simulink model "gm_test_prediction_without_delays"  (R2022a)
settings: Solver=FixedStepDiscrete  StartTime=0.0  StopTime=10.0  RelTol=1e-3
undefined symbols (not defined in the file or in its folder): f_c, L_d, L_q, L_x, L_y, p, psi_pm, R_ph
libraries: hdlmdlgenlib x2
(part 7 of 9)

== system gm_test_prediction_without_delays/Prediction_and_cost_function1/Subsystem/Subsystem12/Add2 ==
  In1 : Inport
  In2 : Inport  Port=2
  Add2 : Sum  OutDataTypeStr=single  SampleTime=1e-08
  Add2_pd1 : Delay  DelayLength=6
  Out1 : Outport
  wires:
  In1/1 -> Add2/1
  In2/1 -> Add2/2
  Add2/1 -> Add2_pd1/1
  Add2_pd1/1 -> Out1/1

== system gm_test_prediction_without_delays/Prediction_and_cost_function1/Subsystem/Subsystem12/Add3 ==
  In1 : Inport
  In2 : Inport  Port=2
  Add3 : Sum  OutDataTypeStr=single  SampleTime=1e-08
  Add3_pd1 : Delay  DelayLength=6
  Out1 : Outport
  wires:
  In1/1 -> Add3/1
  In2/1 -> Add3/2
  Add3/1 -> Add3_pd1/1
  Add3_pd1/1 -> Out1/1

== system gm_test_prediction_without_delays/Prediction_and_cost_function1/Subsystem/Subsystem12/Add4 ==
  In1 : Inport
  In2 : Inport  Port=2
  Add4 : Sum  OutDataTypeStr=single  SampleTime=1e-08
  Add4_pd1 : Delay  DelayLength=6
  Out1 : Outport
  wires:
  In1/1 -> Add4/1
  In2/1 -> Add4/2
  Add4/1 -> Add4_pd1/1
  Add4_pd1/1 -> Out1/1

== system gm_test_prediction_without_delays/Prediction_and_cost_function1/Subsystem/Subsystem12/Product1 ==
  In1 : Inport
  In2 : Inport  Port=2
  Product1 : Product  Inputs=**  OutDataTypeStr=single  SampleTime=1e-08
  Product1_pd1 : Delay  DelayLength=6
  Out1 : Outport
  wires:
  In1/1 -> Product1/1
  In2/1 -> Product1/2
  Product1/1 -> Product1_pd1/1
  Product1_pd1/1 -> Out1/1

== system gm_test_prediction_without_delays/Prediction_and_cost_function1/Subsystem/Subsystem12/Product10 ==
  In1 : Inport
  In2 : Inport  Port=2
  Product10 : Product  Inputs=**  OutDataTypeStr=single  SampleTime=1e-08
  Product10_pd1 : Delay  DelayLength=6
  Out1 : Outport
  wires:
  In1/1 -> Product10/1
  In2/1 -> Product10/2
  Product10/1 -> Product10_pd1/1
  Product10_pd1/1 -> Out1/1

== system gm_test_prediction_without_delays/Prediction_and_cost_function1/Subsystem/Subsystem12/Product11 ==
  In1 : Inport
  In2 : Inport  Port=2
  Product11 : Product  Inputs=**  OutDataTypeStr=single  SampleTime=1e-08
  Product11_pd1 : Delay  DelayLength=6
  Out1 : Outport
  wires:
  In1/1 -> Product11/1
  In2/1 -> Product11/2
  Product11/1 -> Product11_pd1/1
  Product11_pd1/1 -> Out1/1

== system gm_test_prediction_without_delays/Prediction_and_cost_function1/Subsystem/Subsystem12/Product2 ==
  In1 : Inport
  In2 : Inport  Port=2
  Product2 : Product  Inputs=**  OutDataTypeStr=single  SampleTime=1e-08
  Product2_pd1 : Delay  DelayLength=6
  Out1 : Outport
  wires:
  In1/1 -> Product2/1
  In2/1 -> Product2/2
  Product2/1 -> Product2_pd1/1
  Product2_pd1/1 -> Out1/1

== system gm_test_prediction_without_delays/Prediction_and_cost_function1/Subsystem/Subsystem12/Product3 ==
  In1 : Inport
  In2 : Inport  Port=2
  Product3 : Product  Inputs=**  OutDataTypeStr=single  SampleTime=1e-08
  Product3_pd1 : Delay  DelayLength=6
  Out1 : Outport
  wires:
  In1/1 -> Product3/1
  In2/1 -> Product3/2
  Product3/1 -> Product3_pd1/1
  Product3_pd1/1 -> Out1/1

== system gm_test_prediction_without_delays/Prediction_and_cost_function1/Subsystem/Subsystem12/Product31 ==
  In1 : Inport
  In2 : Inport  Port=2
  Product31 : Product  Inputs=**  OutDataTypeStr=single  SampleTime=1e-08
  Product31_pd1 : Delay  DelayLength=6
  Out1 : Outport
  wires:
  In1/1 -> Product31/1
  In2/1 -> Product31/2
  Product31/1 -> Product31_pd1/1
  Product31_pd1/1 -> Out1/1

== system gm_test_prediction_without_delays/Prediction_and_cost_function1/Subsystem/Subsystem12/Product4 ==
  In1 : Inport
  In2 : Inport  Port=2
  Product4 : Product  Inputs=**  OutDataTypeStr=single  SampleTime=1e-08
  Product4_pd1 : Delay  DelayLength=6
  Out1 : Outport
  wires:
  In1/1 -> Product4/1
  In2/1 -> Product4/2
  Product4/1 -> Product4_pd1/1
  Product4_pd1/1 -> Out1/1

== system gm_test_prediction_without_delays/Prediction_and_cost_function1/Subsystem/Subsystem12/Product5 ==
  In1 : Inport
  In2 : Inport  Port=2
  Product5 : Product  Inputs=**  OutDataTypeStr=single  SampleTime=1e-08
  Product5_pd1 : Delay  DelayLength=6
  Out1 : Outport
  wires:
  In1/1 -> Product5/1
  In2/1 -> Product5/2
  Product5/1 -> Product5_pd1/1
  Product5_pd1/1 -> Out1/1

== system gm_test_prediction_without_delays/Prediction_and_cost_function1/Subsystem/Subsystem12/Product6 ==
  In1 : Inport
  In2 : Inport  Port=2
  Product6 : Product  Inputs=**  OutDataTypeStr=single  SampleTime=1e-08
  Product6_pd1 : Delay  DelayLength=6
  Out1 : Outport
  wires:
  In1/1 -> Product6/1
  In2/1 -> Product6/2
  Product6/1 -> Product6_pd1/1
  Product6_pd1/1 -> Out1/1

== system gm_test_prediction_without_delays/Prediction_and_cost_function1/Subsystem/Subsystem12/Product7 ==
  In1 : Inport
  In2 : Inport  Port=2
  Product7 : Product  Inputs=**  OutDataTypeStr=single  SampleTime=1e-08
  Product7_pd1 : Delay  DelayLength=6
  Out1 : Outport
  wires:
  In1/1 -> Product7/1
  In2/1 -> Product7/2
  Product7/1 -> Product7_pd1/1
  Product7_pd1/1 -> Out1/1

== system gm_test_prediction_without_delays/Prediction_and_cost_function1/Subsystem/Subsystem12/Product8 ==
  In1 : Inport
  In2 : Inport  Port=2
  Product8 : Product  Inputs=**  OutDataTypeStr=single  SampleTime=1e-08
  Product8_pd1 : Delay  DelayLength=6
  Out1 : Outport
  wires:
  In1/1 -> Product8/1
  In2/1 -> Product8/2
  Product8/1 -> Product8_pd1/1
  Product8_pd1/1 -> Out1/1

== system gm_test_prediction_without_delays/Prediction_and_cost_function1/Subsystem/Subsystem12/Product9 ==
  In1 : Inport
  In2 : Inport  Port=2
  Product9 : Product  Inputs=**  OutDataTypeStr=single  SampleTime=1e-08
  Product9_pd1 : Delay  DelayLength=6
  Out1 : Outport
  wires:
  In1/1 -> Product9/1
  In2/1 -> Product9/2
  Product9/1 -> Product9_pd1/1
  Product9_pd1/1 -> Out1/1

== system gm_test_prediction_without_delays/Prediction_and_cost_function1/Subsystem/Subsystem12/Subtract1_stage2 ==
  In1 : Inport
  In2 : Inport  Port=2
  Subtract1_stage2 : Sum  Inputs=+-  OutDataTypeStr=single  SampleTime=1e-08
  Subtract1_stage2_pd1 : Delay  DelayLength=6
  Out1 : Outport
  wires:
  In1/1 -> Subtract1_stage2/1
  In2/1 -> Subtract1_stage2/2
  Subtract1_stage2/1 -> Subtract1_stage2_pd1/1
  Subtract1_stage2_pd1/1 -> Out1/1

== system gm_test_prediction_without_delays/Prediction_and_cost_function1/Subsystem/Subsystem12/Subtract1_stage3 ==
  In1 : Inport
  In2 : Inport  Port=2
  Subtract1_stage3 : Sum  Inputs=+-  OutDataTypeStr=single  SampleTime=1e-08
  Subtract1_stage3_pd1 : Delay  DelayLength=6
  Out1 : Outport
  wires:
  In1/1 -> Subtract1_stage3/1
  In2/1 -> Subtract1_stage3/2
  Subtract1_stage3/1 -> Subtract1_stage3_pd1/1
  Subtract1_stage3_pd1/1 -> Out1/1

== system gm_test_prediction_without_delays/Prediction_and_cost_function1/Subsystem/Subsystem12/Subtract2 ==
  In1 : Inport
  In2 : Inport  Port=2
  Subtract2 : Sum  Inputs=+-  OutDataTypeStr=single  SampleTime=1e-08
  Subtract2_pd1 : Delay  DelayLength=6
  Out1 : Outport
  wires:
  In1/1 -> Subtract2/1
  In2/1 -> Subtract2/2
  Subtract2/1 -> Subtract2_pd1/1
  Subtract2_pd1/1 -> Out1/1

== system gm_test_prediction_without_delays/Prediction_and_cost_function1/Subsystem/Subsystem12/Subtract3 ==
  In1 : Inport
  In2 : Inport  Port=2
  Subtract3 : Sum  Inputs=+-  OutDataTypeStr=single  SampleTime=1e-08
  Subtract3_pd1 : Delay  DelayLength=6
  Out1 : Outport
  wires:
  In1/1 -> Subtract3/1
  In2/1 -> Subtract3/2
  Subtract3/1 -> Subtract3_pd1/1
  Subtract3_pd1/1 -> Out1/1

== system gm_test_prediction_without_delays/Prediction_and_cost_function1/Subsystem/Subsystem12/Subtract_stage2 ==
  In1 : Inport
  In2 : Inport  Port=2
  Subtract_stage2 : Sum  Inputs=+-  OutDataTypeStr=single  SampleTime=1e-08
  Subtract_stage2_pd1 : Delay  DelayLength=6
  Out1 : Outport
  wires:
  In1/1 -> Subtract_stage2/1
  In2/1 -> Subtract_stage2/2
  Subtract_stage2/1 -> Subtract_stage2_pd1/1
  Subtract_stage2_pd1/1 -> Out1/1

== system gm_test_prediction_without_delays/Prediction_and_cost_function1/Subsystem/Subsystem12/Subtract_stage3 ==
  In1 : Inport
  In2 : Inport  Port=2
  Subtract_stage3 : Sum  OutDataTypeStr=single  SampleTime=1e-08
  Subtract_stage3_pd1 : Delay  DelayLength=6
  Out1 : Outport
  wires:
  In1/1 -> Subtract_stage3/1
  In2/1 -> Subtract_stage3/2
  Subtract_stage3/1 -> Subtract_stage3_pd1/1
  Subtract_stage3_pd1/1 -> Out1/1

== system gm_test_prediction_without_delays/Prediction_and_cost_function1/Subsystem/Subsystem13/Add ==
  In1 : Inport
  In2 : Inport  Port=2
  Add : Sum  OutDataTypeStr=single  SampleTime=1e-08
  Add_pd1 : Delay  DelayLength=6
  Out1 : Outport
  wires:
  In1/1 -> Add/1
  In2/1 -> Add/2
  Add/1 -> Add_pd1/1
  Add_pd1/1 -> Out1/1

== system gm_test_prediction_without_delays/Prediction_and_cost_function1/Subsystem/Subsystem13/Add1 ==
  In1 : Inport
  In2 : Inport  Port=2
  Add1 : Sum  OutDataTypeStr=single  SampleTime=1e-08
  Add1_pd1 : Delay  DelayLength=6
  Out1 : Outport
  wires:
  In1/1 -> Add1/1
  In2/1 -> Add1/2
  Add1/1 -> Add1_pd1/1
  Add1_pd1/1 -> Out1/1

== system gm_test_prediction_without_delays/Prediction_and_cost_function1/Subsystem/Subsystem13/Add2 ==
  In1 : Inport
  In2 : Inport  Port=2
  Add2 : Sum  OutDataTypeStr=single  SampleTime=1e-08
  Add2_pd1 : Delay  DelayLength=6
  Out1 : Outport
  wires:
  In1/1 -> Add2/1
  In2/1 -> Add2/2
  Add2/1 -> Add2_pd1/1
  Add2_pd1/1 -> Out1/1

== system gm_test_prediction_without_delays/Prediction_and_cost_function1/Subsystem/Subsystem13/Add3 ==
  In1 : Inport
  In2 : Inport  Port=2
  Add3 : Sum  OutDataTypeStr=single  SampleTime=1e-08
  Add3_pd1 : Delay  DelayLength=6
  Out1 : Outport
  wires:
  In1/1 -> Add3/1
  In2/1 -> Add3/2
  Add3/1 -> Add3_pd1/1
  Add3_pd1/1 -> Out1/1

== system gm_test_prediction_without_delays/Prediction_and_cost_function1/Subsystem/Subsystem13/Add4 ==
  In1 : Inport
  In2 : Inport  Port=2
  Add4 : Sum  OutDataTypeStr=single  SampleTime=1e-08
  Add4_pd1 : Delay  DelayLength=6
  Out1 : Outport
  wires:
  In1/1 -> Add4/1
  In2/1 -> Add4/2
  Add4/1 -> Add4_pd1/1
  Add4_pd1/1 -> Out1/1

== system gm_test_prediction_without_delays/Prediction_and_cost_function1/Subsystem/Subsystem13/Product1 ==
  In1 : Inport
  In2 : Inport  Port=2
  Product1 : Product  Inputs=**  OutDataTypeStr=single  SampleTime=1e-08
  Product1_pd1 : Delay  DelayLength=6
  Out1 : Outport
  wires:
  In1/1 -> Product1/1
  In2/1 -> Product1/2
  Product1/1 -> Product1_pd1/1
  Product1_pd1/1 -> Out1/1

== system gm_test_prediction_without_delays/Prediction_and_cost_function1/Subsystem/Subsystem13/Product10 ==
  In1 : Inport
  In2 : Inport  Port=2
  Product10 : Product  Inputs=**  OutDataTypeStr=single  SampleTime=1e-08
  Product10_pd1 : Delay  DelayLength=6
  Out1 : Outport
  wires:
  In1/1 -> Product10/1
  In2/1 -> Product10/2
  Product10/1 -> Product10_pd1/1
  Product10_pd1/1 -> Out1/1

== system gm_test_prediction_without_delays/Prediction_and_cost_function1/Subsystem/Subsystem13/Product11 ==
  In1 : Inport
  In2 : Inport  Port=2
  Product11 : Product  Inputs=**  OutDataTypeStr=single  SampleTime=1e-08
  Product11_pd1 : Delay  DelayLength=6
  Out1 : Outport
  wires:
  In1/1 -> Product11/1
  In2/1 -> Product11/2
  Product11/1 -> Product11_pd1/1
  Product11_pd1/1 -> Out1/1

== system gm_test_prediction_without_delays/Prediction_and_cost_function1/Subsystem/Subsystem13/Product2 ==
  In1 : Inport
  In2 : Inport  Port=2
  Product2 : Product  Inputs=**  OutDataTypeStr=single  SampleTime=1e-08
  Product2_pd1 : Delay  DelayLength=6
  Out1 : Outport
  wires:
  In1/1 -> Product2/1
  In2/1 -> Product2/2
  Product2/1 -> Product2_pd1/1
  Product2_pd1/1 -> Out1/1

== system gm_test_prediction_without_delays/Prediction_and_cost_function1/Subsystem/Subsystem13/Product3 ==
  In1 : Inport
  In2 : Inport  Port=2
  Product3 : Product  Inputs=**  OutDataTypeStr=single  SampleTime=1e-08
  Product3_pd1 : Delay  DelayLength=6
  Out1 : Outport
  wires:
  In1/1 -> Product3/1
  In2/1 -> Product3/2
  Product3/1 -> Product3_pd1/1
  Product3_pd1/1 -> Out1/1

== system gm_test_prediction_without_delays/Prediction_and_cost_function1/Subsystem/Subsystem13/Product31 ==
  In1 : Inport
  In2 : Inport  Port=2
  Product31 : Product  Inputs=**  OutDataTypeStr=single  SampleTime=1e-08
  Product31_pd1 : Delay  DelayLength=6
  Out1 : Outport
  wires:
  In1/1 -> Product31/1
  In2/1 -> Product31/2
  Product31/1 -> Product31_pd1/1
  Product31_pd1/1 -> Out1/1

== system gm_test_prediction_without_delays/Prediction_and_cost_function1/Subsystem/Subsystem13/Product4 ==
  In1 : Inport
  In2 : Inport  Port=2
  Product4 : Product  Inputs=**  OutDataTypeStr=single  SampleTime=1e-08
  Product4_pd1 : Delay  DelayLength=6
  Out1 : Outport
  wires:
  In1/1 -> Product4/1
  In2/1 -> Product4/2
  Product4/1 -> Product4_pd1/1
  Product4_pd1/1 -> Out1/1

== system gm_test_prediction_without_delays/Prediction_and_cost_function1/Subsystem/Subsystem13/Product5 ==
  In1 : Inport
  In2 : Inport  Port=2
  Product5 : Product  Inputs=**  OutDataTypeStr=single  SampleTime=1e-08
  Product5_pd1 : Delay  DelayLength=6
  Out1 : Outport
  wires:
  In1/1 -> Product5/1
  In2/1 -> Product5/2
  Product5/1 -> Product5_pd1/1
  Product5_pd1/1 -> Out1/1

== system gm_test_prediction_without_delays/Prediction_and_cost_function1/Subsystem/Subsystem13/Product6 ==
  In1 : Inport
  In2 : Inport  Port=2
  Product6 : Product  Inputs=**  OutDataTypeStr=single  SampleTime=1e-08
  Product6_pd1 : Delay  DelayLength=6
  Out1 : Outport
  wires:
  In1/1 -> Product6/1
  In2/1 -> Product6/2
  Product6/1 -> Product6_pd1/1
  Product6_pd1/1 -> Out1/1

== system gm_test_prediction_without_delays/Prediction_and_cost_function1/Subsystem/Subsystem13/Product7 ==
  In1 : Inport
  In2 : Inport  Port=2
  Product7 : Product  Inputs=**  OutDataTypeStr=single  SampleTime=1e-08
  Product7_pd1 : Delay  DelayLength=6
  Out1 : Outport
  wires:
  In1/1 -> Product7/1
  In2/1 -> Product7/2
  Product7/1 -> Product7_pd1/1
  Product7_pd1/1 -> Out1/1

== system gm_test_prediction_without_delays/Prediction_and_cost_function1/Subsystem/Subsystem13/Product8 ==
  In1 : Inport
  In2 : Inport  Port=2
  Product8 : Product  Inputs=**  OutDataTypeStr=single  SampleTime=1e-08
  Product8_pd1 : Delay  DelayLength=6
  Out1 : Outport
  wires:
  In1/1 -> Product8/1
  In2/1 -> Product8/2
  Product8/1 -> Product8_pd1/1
  Product8_pd1/1 -> Out1/1

== system gm_test_prediction_without_delays/Prediction_and_cost_function1/Subsystem/Subsystem13/Product9 ==
  In1 : Inport
  In2 : Inport  Port=2
  Product9 : Product  Inputs=**  OutDataTypeStr=single  SampleTime=1e-08
  Product9_pd1 : Delay  DelayLength=6
  Out1 : Outport
  wires:
  In1/1 -> Product9/1
  In2/1 -> Product9/2
  Product9/1 -> Product9_pd1/1
  Product9_pd1/1 -> Out1/1

== system gm_test_prediction_without_delays/Prediction_and_cost_function1/Subsystem/Subsystem13/Subtract1_stage2 ==
  In1 : Inport
  In2 : Inport  Port=2
  Subtract1_stage2 : Sum  Inputs=+-  OutDataTypeStr=single  SampleTime=1e-08
  Subtract1_stage2_pd1 : Delay  DelayLength=6
  Out1 : Outport
  wires:
  In1/1 -> Subtract1_stage2/1
  In2/1 -> Subtract1_stage2/2
  Subtract1_stage2/1 -> Subtract1_stage2_pd1/1
  Subtract1_stage2_pd1/1 -> Out1/1

== system gm_test_prediction_without_delays/Prediction_and_cost_function1/Subsystem/Subsystem13/Subtract1_stage3 ==
  In1 : Inport
  In2 : Inport  Port=2
  Subtract1_stage3 : Sum  Inputs=+-  OutDataTypeStr=single  SampleTime=1e-08
  Subtract1_stage3_pd1 : Delay  DelayLength=6
  Out1 : Outport
  wires:
  In1/1 -> Subtract1_stage3/1
  In2/1 -> Subtract1_stage3/2
  Subtract1_stage3/1 -> Subtract1_stage3_pd1/1
  Subtract1_stage3_pd1/1 -> Out1/1

== system gm_test_prediction_without_delays/Prediction_and_cost_function1/Subsystem/Subsystem13/Subtract2 ==
  In1 : Inport
  In2 : Inport  Port=2
  Subtract2 : Sum  Inputs=+-  OutDataTypeStr=single  SampleTime=1e-08
  Subtract2_pd1 : Delay  DelayLength=6
  Out1 : Outport
  wires:
  In1/1 -> Subtract2/1
  In2/1 -> Subtract2/2
  Subtract2/1 -> Subtract2_pd1/1
  Subtract2_pd1/1 -> Out1/1

== system gm_test_prediction_without_delays/Prediction_and_cost_function1/Subsystem/Subsystem13/Subtract3 ==
  In1 : Inport
  In2 : Inport  Port=2
  Subtract3 : Sum  Inputs=+-  OutDataTypeStr=single  SampleTime=1e-08
  Subtract3_pd1 : Delay  DelayLength=6
  Out1 : Outport
  wires:
  In1/1 -> Subtract3/1
  In2/1 -> Subtract3/2
  Subtract3/1 -> Subtract3_pd1/1
  Subtract3_pd1/1 -> Out1/1

== system gm_test_prediction_without_delays/Prediction_and_cost_function1/Subsystem/Subsystem13/Subtract_stage2 ==
  In1 : Inport
  In2 : Inport  Port=2
  Subtract_stage2 : Sum  Inputs=+-  OutDataTypeStr=single  SampleTime=1e-08
  Subtract_stage2_pd1 : Delay  DelayLength=6
  Out1 : Outport
  wires:
  In1/1 -> Subtract_stage2/1
  In2/1 -> Subtract_stage2/2
  Subtract_stage2/1 -> Subtract_stage2_pd1/1
  Subtract_stage2_pd1/1 -> Out1/1

== system gm_test_prediction_without_delays/Prediction_and_cost_function1/Subsystem/Subsystem13/Subtract_stage3 ==
  In1 : Inport
  In2 : Inport  Port=2
  Subtract_stage3 : Sum  OutDataTypeStr=single  SampleTime=1e-08
  Subtract_stage3_pd1 : Delay  DelayLength=6
  Out1 : Outport
  wires:
  In1/1 -> Subtract_stage3/1
  In2/1 -> Subtract_stage3/2
  Subtract_stage3/1 -> Subtract_stage3_pd1/1
  Subtract_stage3_pd1/1 -> Out1/1

== system gm_test_prediction_without_delays/Prediction_and_cost_function1/Subsystem/Subsystem14/Add ==
  In1 : Inport
  In2 : Inport  Port=2
  Add : Sum  OutDataTypeStr=single  SampleTime=1e-08
  Add_pd1 : Delay  DelayLength=6
  Out1 : Outport
  wires:
  In1/1 -> Add/1
  In2/1 -> Add/2
  Add/1 -> Add_pd1/1
  Add_pd1/1 -> Out1/1

== system gm_test_prediction_without_delays/Prediction_and_cost_function1/Subsystem/Subsystem14/Add1 ==
  In1 : Inport
  In2 : Inport  Port=2
  Add1 : Sum  OutDataTypeStr=single  SampleTime=1e-08
  Add1_pd1 : Delay  DelayLength=6
  Out1 : Outport
  wires:
  In1/1 -> Add1/1
  In2/1 -> Add1/2
  Add1/1 -> Add1_pd1/1
  Add1_pd1/1 -> Out1/1

== system gm_test_prediction_without_delays/Prediction_and_cost_function1/Subsystem/Subsystem14/Add2 ==
  In1 : Inport
  In2 : Inport  Port=2
  Add2 : Sum  OutDataTypeStr=single  SampleTime=1e-08
  Add2_pd1 : Delay  DelayLength=6
  Out1 : Outport
  wires:
  In1/1 -> Add2/1
  In2/1 -> Add2/2
  Add2/1 -> Add2_pd1/1
  Add2_pd1/1 -> Out1/1

== system gm_test_prediction_without_delays/Prediction_and_cost_function1/Subsystem/Subsystem14/Add3 ==
  In1 : Inport
  In2 : Inport  Port=2
  Add3 : Sum  OutDataTypeStr=single  SampleTime=1e-08
  Add3_pd1 : Delay  DelayLength=6
  Out1 : Outport
  wires:
  In1/1 -> Add3/1
  In2/1 -> Add3/2
  Add3/1 -> Add3_pd1/1
  Add3_pd1/1 -> Out1/1

== system gm_test_prediction_without_delays/Prediction_and_cost_function1/Subsystem/Subsystem14/Add4 ==
  In1 : Inport
  In2 : Inport  Port=2
  Add4 : Sum  OutDataTypeStr=single  SampleTime=1e-08
  Add4_pd1 : Delay  DelayLength=6
  Out1 : Outport
  wires:
  In1/1 -> Add4/1
  In2/1 -> Add4/2
  Add4/1 -> Add4_pd1/1
  Add4_pd1/1 -> Out1/1

== system gm_test_prediction_without_delays/Prediction_and_cost_function1/Subsystem/Subsystem14/Product1 ==
  In1 : Inport
  In2 : Inport  Port=2
  Product1 : Product  Inputs=**  OutDataTypeStr=single  SampleTime=1e-08
  Product1_pd1 : Delay  DelayLength=6
  Out1 : Outport
  wires:
  In1/1 -> Product1/1
  In2/1 -> Product1/2
  Product1/1 -> Product1_pd1/1
  Product1_pd1/1 -> Out1/1

== system gm_test_prediction_without_delays/Prediction_and_cost_function1/Subsystem/Subsystem14/Product10 ==
  In1 : Inport
  In2 : Inport  Port=2
  Product10 : Product  Inputs=**  OutDataTypeStr=single  SampleTime=1e-08
  Product10_pd1 : Delay  DelayLength=6
  Out1 : Outport
  wires:
  In1/1 -> Product10/1
  In2/1 -> Product10/2
  Product10/1 -> Product10_pd1/1
  Product10_pd1/1 -> Out1/1

== system gm_test_prediction_without_delays/Prediction_and_cost_function1/Subsystem/Subsystem14/Product11 ==
  In1 : Inport
  In2 : Inport  Port=2
  Product11 : Product  Inputs=**  OutDataTypeStr=single  SampleTime=1e-08
  Product11_pd1 : Delay  DelayLength=6
  Out1 : Outport
  wires:
  In1/1 -> Product11/1
  In2/1 -> Product11/2
  Product11/1 -> Product11_pd1/1
  Product11_pd1/1 -> Out1/1

== system gm_test_prediction_without_delays/Prediction_and_cost_function1/Subsystem/Subsystem14/Product2 ==
  In1 : Inport
  In2 : Inport  Port=2
  Product2 : Product  Inputs=**  OutDataTypeStr=single  SampleTime=1e-08
  Product2_pd1 : Delay  DelayLength=6
  Out1 : Outport
  wires:
  In1/1 -> Product2/1
  In2/1 -> Product2/2
  Product2/1 -> Product2_pd1/1
  Product2_pd1/1 -> Out1/1

== system gm_test_prediction_without_delays/Prediction_and_cost_function1/Subsystem/Subsystem14/Product3 ==
  In1 : Inport
  In2 : Inport  Port=2
  Product3 : Product  Inputs=**  OutDataTypeStr=single  SampleTime=1e-08
  Product3_pd1 : Delay  DelayLength=6
  Out1 : Outport
  wires:
  In1/1 -> Product3/1
  In2/1 -> Product3/2
  Product3/1 -> Product3_pd1/1
  Product3_pd1/1 -> Out1/1

== system gm_test_prediction_without_delays/Prediction_and_cost_function1/Subsystem/Subsystem14/Product31 ==
  In1 : Inport
  In2 : Inport  Port=2
  Product31 : Product  Inputs=**  OutDataTypeStr=single  SampleTime=1e-08
  Product31_pd1 : Delay  DelayLength=6
  Out1 : Outport
  wires:
  In1/1 -> Product31/1
  In2/1 -> Product31/2
  Product31/1 -> Product31_pd1/1
  Product31_pd1/1 -> Out1/1

== system gm_test_prediction_without_delays/Prediction_and_cost_function1/Subsystem/Subsystem14/Product4 ==
  In1 : Inport
  In2 : Inport  Port=2
  Product4 : Product  Inputs=**  OutDataTypeStr=single  SampleTime=1e-08
  Product4_pd1 : Delay  DelayLength=6
  Out1 : Outport
  wires:
  In1/1 -> Product4/1
  In2/1 -> Product4/2
  Product4/1 -> Product4_pd1/1
  Product4_pd1/1 -> Out1/1

== system gm_test_prediction_without_delays/Prediction_and_cost_function1/Subsystem/Subsystem14/Product5 ==
  In1 : Inport
  In2 : Inport  Port=2
  Product5 : Product  Inputs=**  OutDataTypeStr=single  SampleTime=1e-08
  Product5_pd1 : Delay  DelayLength=6
  Out1 : Outport
  wires:
  In1/1 -> Product5/1
  In2/1 -> Product5/2
  Product5/1 -> Product5_pd1/1
  Product5_pd1/1 -> Out1/1

== system gm_test_prediction_without_delays/Prediction_and_cost_function1/Subsystem/Subsystem14/Product6 ==
  In1 : Inport
  In2 : Inport  Port=2
  Product6 : Product  Inputs=**  OutDataTypeStr=single  SampleTime=1e-08
  Product6_pd1 : Delay  DelayLength=6
  Out1 : Outport
  wires:
  In1/1 -> Product6/1
  In2/1 -> Product6/2
  Product6/1 -> Product6_pd1/1
  Product6_pd1/1 -> Out1/1

== system gm_test_prediction_without_delays/Prediction_and_cost_function1/Subsystem/Subsystem14/Product7 ==
  In1 : Inport
  In2 : Inport  Port=2
  Product7 : Product  Inputs=**  OutDataTypeStr=single  SampleTime=1e-08
  Product7_pd1 : Delay  DelayLength=6
  Out1 : Outport
  wires:
  In1/1 -> Product7/1
  In2/1 -> Product7/2
  Product7/1 -> Product7_pd1/1
  Product7_pd1/1 -> Out1/1

== system gm_test_prediction_without_delays/Prediction_and_cost_function1/Subsystem/Subsystem14/Product8 ==
  In1 : Inport
  In2 : Inport  Port=2
  Product8 : Product  Inputs=**  OutDataTypeStr=single  SampleTime=1e-08
  Product8_pd1 : Delay  DelayLength=6
  Out1 : Outport
  wires:
  In1/1 -> Product8/1
  In2/1 -> Product8/2
  Product8/1 -> Product8_pd1/1
  Product8_pd1/1 -> Out1/1

== system gm_test_prediction_without_delays/Prediction_and_cost_function1/Subsystem/Subsystem14/Product9 ==
  In1 : Inport
  In2 : Inport  Port=2
  Product9 : Product  Inputs=**  OutDataTypeStr=single  SampleTime=1e-08
  Product9_pd1 : Delay  DelayLength=6
  Out1 : Outport
  wires:
  In1/1 -> Product9/1
  In2/1 -> Product9/2
  Product9/1 -> Product9_pd1/1
  Product9_pd1/1 -> Out1/1

== system gm_test_prediction_without_delays/Prediction_and_cost_function1/Subsystem/Subsystem14/Subtract1_stage2 ==
  In1 : Inport
  In2 : Inport  Port=2
  Subtract1_stage2 : Sum  Inputs=+-  OutDataTypeStr=single  SampleTime=1e-08
  Subtract1_stage2_pd1 : Delay  DelayLength=6
  Out1 : Outport
  wires:
  In1/1 -> Subtract1_stage2/1
  In2/1 -> Subtract1_stage2/2
  Subtract1_stage2/1 -> Subtract1_stage2_pd1/1
  Subtract1_stage2_pd1/1 -> Out1/1

== system gm_test_prediction_without_delays/Prediction_and_cost_function1/Subsystem/Subsystem14/Subtract1_stage3 ==
  In1 : Inport
  In2 : Inport  Port=2
  Subtract1_stage3 : Sum  Inputs=+-  OutDataTypeStr=single  SampleTime=1e-08
  Subtract1_stage3_pd1 : Delay  DelayLength=6
  Out1 : Outport
  wires:
  In1/1 -> Subtract1_stage3/1
  In2/1 -> Subtract1_stage3/2
  Subtract1_stage3/1 -> Subtract1_stage3_pd1/1
  Subtract1_stage3_pd1/1 -> Out1/1

== system gm_test_prediction_without_delays/Prediction_and_cost_function1/Subsystem/Subsystem14/Subtract2 ==
  In1 : Inport
  In2 : Inport  Port=2
  Subtract2 : Sum  Inputs=+-  OutDataTypeStr=single  SampleTime=1e-08
  Subtract2_pd1 : Delay  DelayLength=6
  Out1 : Outport
  wires:
  In1/1 -> Subtract2/1
  In2/1 -> Subtract2/2
  Subtract2/1 -> Subtract2_pd1/1
  Subtract2_pd1/1 -> Out1/1

== system gm_test_prediction_without_delays/Prediction_and_cost_function1/Subsystem/Subsystem14/Subtract3 ==
  In1 : Inport
  In2 : Inport  Port=2
  Subtract3 : Sum  Inputs=+-  OutDataTypeStr=single  SampleTime=1e-08
  Subtract3_pd1 : Delay  DelayLength=6
  Out1 : Outport
  wires:
  In1/1 -> Subtract3/1
  In2/1 -> Subtract3/2
  Subtract3/1 -> Subtract3_pd1/1
  Subtract3_pd1/1 -> Out1/1

== system gm_test_prediction_without_delays/Prediction_and_cost_function1/Subsystem/Subsystem14/Subtract_stage2 ==
  In1 : Inport
  In2 : Inport  Port=2
  Subtract_stage2 : Sum  Inputs=+-  OutDataTypeStr=single  SampleTime=1e-08
  Subtract_stage2_pd1 : Delay  DelayLength=6
  Out1 : Outport
  wires:
  In1/1 -> Subtract_stage2/1
  In2/1 -> Subtract_stage2/2
  Subtract_stage2/1 -> Subtract_stage2_pd1/1
  Subtract_stage2_pd1/1 -> Out1/1

== system gm_test_prediction_without_delays/Prediction_and_cost_function1/Subsystem/Subsystem14/Subtract_stage3 ==
  In1 : Inport
  In2 : Inport  Port=2
  Subtract_stage3 : Sum  OutDataTypeStr=single  SampleTime=1e-08
  Subtract_stage3_pd1 : Delay  DelayLength=6
  Out1 : Outport
  wires:
  In1/1 -> Subtract_stage3/1
  In2/1 -> Subtract_stage3/2
  Subtract_stage3/1 -> Subtract_stage3_pd1/1
  Subtract_stage3_pd1/1 -> Out1/1

== system gm_test_prediction_without_delays/Prediction_and_cost_function1/Subsystem/Subsystem15/Add ==
  In1 : Inport
  In2 : Inport  Port=2
  Add : Sum  OutDataTypeStr=single  SampleTime=1e-08
  Add_pd1 : Delay  DelayLength=6
  Out1 : Outport
  wires:
  In1/1 -> Add/1
  In2/1 -> Add/2
  Add/1 -> Add_pd1/1
  Add_pd1/1 -> Out1/1

== system gm_test_prediction_without_delays/Prediction_and_cost_function1/Subsystem/Subsystem15/Add1 ==
  In1 : Inport
  In2 : Inport  Port=2
  Add1 : Sum  OutDataTypeStr=single  SampleTime=1e-08
  Add1_pd1 : Delay  DelayLength=6
  Out1 : Outport
  wires:
  In1/1 -> Add1/1
  In2/1 -> Add1/2
  Add1/1 -> Add1_pd1/1
  Add1_pd1/1 -> Out1/1

== system gm_test_prediction_without_delays/Prediction_and_cost_function1/Subsystem/Subsystem15/Add2 ==
  In1 : Inport
  In2 : Inport  Port=2
  Add2 : Sum  OutDataTypeStr=single  SampleTime=1e-08
  Add2_pd1 : Delay  DelayLength=6
  Out1 : Outport
  wires:
  In1/1 -> Add2/1
  In2/1 -> Add2/2
  Add2/1 -> Add2_pd1/1
  Add2_pd1/1 -> Out1/1

== system gm_test_prediction_without_delays/Prediction_and_cost_function1/Subsystem/Subsystem15/Add3 ==
  In1 : Inport
  In2 : Inport  Port=2
  Add3 : Sum  OutDataTypeStr=single  SampleTime=1e-08
  Add3_pd1 : Delay  DelayLength=6
  Out1 : Outport
  wires:
  In1/1 -> Add3/1
  In2/1 -> Add3/2
  Add3/1 -> Add3_pd1/1
  Add3_pd1/1 -> Out1/1

== system gm_test_prediction_without_delays/Prediction_and_cost_function1/Subsystem/Subsystem15/Add4 ==
  In1 : Inport
  In2 : Inport  Port=2
  Add4 : Sum  OutDataTypeStr=single  SampleTime=1e-08
  Add4_pd1 : Delay  DelayLength=6
  Out1 : Outport
  wires:
  In1/1 -> Add4/1
  In2/1 -> Add4/2
  Add4/1 -> Add4_pd1/1
  Add4_pd1/1 -> Out1/1

== system gm_test_prediction_without_delays/Prediction_and_cost_function1/Subsystem/Subsystem15/Product1 ==
  In1 : Inport
  In2 : Inport  Port=2
  Product1 : Product  Inputs=**  OutDataTypeStr=single  SampleTime=1e-08
  Product1_pd1 : Delay  DelayLength=6
  Out1 : Outport
  wires:
  In1/1 -> Product1/1
  In2/1 -> Product1/2
  Product1/1 -> Product1_pd1/1
  Product1_pd1/1 -> Out1/1

== system gm_test_prediction_without_delays/Prediction_and_cost_function1/Subsystem/Subsystem15/Product10 ==
  In1 : Inport
  In2 : Inport  Port=2
  Product10 : Product  Inputs=**  OutDataTypeStr=single  SampleTime=1e-08
  Product10_pd1 : Delay  DelayLength=6
  Out1 : Outport
  wires:
  In1/1 -> Product10/1
  In2/1 -> Product10/2
  Product10/1 -> Product10_pd1/1
  Product10_pd1/1 -> Out1/1

== system gm_test_prediction_without_delays/Prediction_and_cost_function1/Subsystem/Subsystem15/Product11 ==
  In1 : Inport
  In2 : Inport  Port=2
  Product11 : Product  Inputs=**  OutDataTypeStr=single  SampleTime=1e-08
  Product11_pd1 : Delay  DelayLength=6
  Out1 : Outport
  wires:
  In1/1 -> Product11/1
  In2/1 -> Product11/2
  Product11/1 -> Product11_pd1/1
  Product11_pd1/1 -> Out1/1

== system gm_test_prediction_without_delays/Prediction_and_cost_function1/Subsystem/Subsystem15/Product2 ==
  In1 : Inport
  In2 : Inport  Port=2
  Product2 : Product  Inputs=**  OutDataTypeStr=single  SampleTime=1e-08
  Product2_pd1 : Delay  DelayLength=6
  Out1 : Outport
  wires:
  In1/1 -> Product2/1
  In2/1 -> Product2/2
  Product2/1 -> Product2_pd1/1
  Product2_pd1/1 -> Out1/1

== system gm_test_prediction_without_delays/Prediction_and_cost_function1/Subsystem/Subsystem15/Product3 ==
  In1 : Inport
  In2 : Inport  Port=2
  Product3 : Product  Inputs=**  OutDataTypeStr=single  SampleTime=1e-08
  Product3_pd1 : Delay  DelayLength=6
  Out1 : Outport
  wires:
  In1/1 -> Product3/1
  In2/1 -> Product3/2
  Product3/1 -> Product3_pd1/1
  Product3_pd1/1 -> Out1/1

== system gm_test_prediction_without_delays/Prediction_and_cost_function1/Subsystem/Subsystem15/Product31 ==
  In1 : Inport
  In2 : Inport  Port=2
  Product31 : Product  Inputs=**  OutDataTypeStr=single  SampleTime=1e-08
  Product31_pd1 : Delay  DelayLength=6
  Out1 : Outport
  wires:
  In1/1 -> Product31/1
  In2/1 -> Product31/2
  Product31/1 -> Product31_pd1/1
  Product31_pd1/1 -> Out1/1

== system gm_test_prediction_without_delays/Prediction_and_cost_function1/Subsystem/Subsystem15/Product4 ==
  In1 : Inport
  In2 : Inport  Port=2
  Product4 : Product  Inputs=**  OutDataTypeStr=single  SampleTime=1e-08
  Product4_pd1 : Delay  DelayLength=6
  Out1 : Outport
  wires:
  In1/1 -> Product4/1
  In2/1 -> Product4/2
  Product4/1 -> Product4_pd1/1
  Product4_pd1/1 -> Out1/1

== system gm_test_prediction_without_delays/Prediction_and_cost_function1/Subsystem/Subsystem15/Product5 ==
  In1 : Inport
  In2 : Inport  Port=2
  Product5 : Product  Inputs=**  OutDataTypeStr=single  SampleTime=1e-08
  Product5_pd1 : Delay  DelayLength=6
  Out1 : Outport
  wires:
  In1/1 -> Product5/1
  In2/1 -> Product5/2
  Product5/1 -> Product5_pd1/1
  Product5_pd1/1 -> Out1/1

== system gm_test_prediction_without_delays/Prediction_and_cost_function1/Subsystem/Subsystem15/Product6 ==
  In1 : Inport
  In2 : Inport  Port=2
  Product6 : Product  Inputs=**  OutDataTypeStr=single  SampleTime=1e-08
  Product6_pd1 : Delay  DelayLength=6
  Out1 : Outport
  wires:
  In1/1 -> Product6/1
  In2/1 -> Product6/2
  Product6/1 -> Product6_pd1/1
  Product6_pd1/1 -> Out1/1

== system gm_test_prediction_without_delays/Prediction_and_cost_function1/Subsystem/Subsystem15/Product7 ==
  In1 : Inport
  In2 : Inport  Port=2
  Product7 : Product  Inputs=**  OutDataTypeStr=single  SampleTime=1e-08
  Product7_pd1 : Delay  DelayLength=6
  Out1 : Outport
  wires:
  In1/1 -> Product7/1
  In2/1 -> Product7/2
  Product7/1 -> Product7_pd1/1
  Product7_pd1/1 -> Out1/1

== system gm_test_prediction_without_delays/Prediction_and_cost_function1/Subsystem/Subsystem15/Product8 ==
  In1 : Inport
  In2 : Inport  Port=2
  Product8 : Product  Inputs=**  OutDataTypeStr=single  SampleTime=1e-08
  Product8_pd1 : Delay  DelayLength=6
  Out1 : Outport
  wires:
  In1/1 -> Product8/1
  In2/1 -> Product8/2
  Product8/1 -> Product8_pd1/1
  Product8_pd1/1 -> Out1/1

== system gm_test_prediction_without_delays/Prediction_and_cost_function1/Subsystem/Subsystem15/Product9 ==
  In1 : Inport
  In2 : Inport  Port=2
  Product9 : Product  Inputs=**  OutDataTypeStr=single  SampleTime=1e-08
  Product9_pd1 : Delay  DelayLength=6
  Out1 : Outport
  wires:
  In1/1 -> Product9/1
  In2/1 -> Product9/2
  Product9/1 -> Product9_pd1/1
  Product9_pd1/1 -> Out1/1

== system gm_test_prediction_without_delays/Prediction_and_cost_function1/Subsystem/Subsystem15/Subtract1_stage2 ==
  In1 : Inport
  In2 : Inport  Port=2
  Subtract1_stage2 : Sum  Inputs=+-  OutDataTypeStr=single  SampleTime=1e-08
  Subtract1_stage2_pd1 : Delay  DelayLength=6
  Out1 : Outport
  wires:
  In1/1 -> Subtract1_stage2/1
  In2/1 -> Subtract1_stage2/2
  Subtract1_stage2/1 -> Subtract1_stage2_pd1/1
  Subtract1_stage2_pd1/1 -> Out1/1

== system gm_test_prediction_without_delays/Prediction_and_cost_function1/Subsystem/Subsystem15/Subtract1_stage3 ==
  In1 : Inport
  In2 : Inport  Port=2
  Subtract1_stage3 : Sum  Inputs=+-  OutDataTypeStr=single  SampleTime=1e-08
  Subtract1_stage3_pd1 : Delay  DelayLength=6
  Out1 : Outport
  wires:
  In1/1 -> Subtract1_stage3/1
  In2/1 -> Subtract1_stage3/2
  Subtract1_stage3/1 -> Subtract1_stage3_pd1/1
  Subtract1_stage3_pd1/1 -> Out1/1

== system gm_test_prediction_without_delays/Prediction_and_cost_function1/Subsystem/Subsystem15/Subtract2 ==
  In1 : Inport
  In2 : Inport  Port=2
  Subtract2 : Sum  Inputs=+-  OutDataTypeStr=single  SampleTime=1e-08
  Subtract2_pd1 : Delay  DelayLength=6
  Out1 : Outport
  wires:
  In1/1 -> Subtract2/1
  In2/1 -> Subtract2/2
  Subtract2/1 -> Subtract2_pd1/1
  Subtract2_pd1/1 -> Out1/1

== system gm_test_prediction_without_delays/Prediction_and_cost_function1/Subsystem/Subsystem15/Subtract3 ==
  In1 : Inport
  In2 : Inport  Port=2
  Subtract3 : Sum  Inputs=+-  OutDataTypeStr=single  SampleTime=1e-08
  Subtract3_pd1 : Delay  DelayLength=6
  Out1 : Outport
  wires:
  In1/1 -> Subtract3/1
  In2/1 -> Subtract3/2
  Subtract3/1 -> Subtract3_pd1/1
  Subtract3_pd1/1 -> Out1/1

== system gm_test_prediction_without_delays/Prediction_and_cost_function1/Subsystem/Subsystem15/Subtract_stage2 ==
  In1 : Inport
  In2 : Inport  Port=2
  Subtract_stage2 : Sum  Inputs=+-  OutDataTypeStr=single  SampleTime=1e-08
  Subtract_stage2_pd1 : Delay  DelayLength=6
  Out1 : Outport
  wires:
  In1/1 -> Subtract_stage2/1
  In2/1 -> Subtract_stage2/2
  Subtract_stage2/1 -> Subtract_stage2_pd1/1
  Subtract_stage2_pd1/1 -> Out1/1

== system gm_test_prediction_without_delays/Prediction_and_cost_function1/Subsystem/Subsystem15/Subtract_stage3 ==
  In1 : Inport
  In2 : Inport  Port=2
  Subtract_stage3 : Sum  OutDataTypeStr=single  SampleTime=1e-08
  Subtract_stage3_pd1 : Delay  DelayLength=6
  Out1 : Outport
  wires:
  In1/1 -> Subtract_stage3/1
  In2/1 -> Subtract_stage3/2
  Subtract_stage3/1 -> Subtract_stage3_pd1/1
  Subtract_stage3_pd1/1 -> Out1/1

== system gm_test_prediction_without_delays/Prediction_and_cost_function1/Subsystem/Subsystem2/Add ==
  In1 : Inport
  In2 : Inport  Port=2
  Add : Sum  OutDataTypeStr=single  SampleTime=1e-08
  Add_pd1 : Delay  DelayLength=6
  Out1 : Outport
  wires:
  In1/1 -> Add/1
  In2/1 -> Add/2
  Add/1 -> Add_pd1/1
  Add_pd1/1 -> Out1/1

== system gm_test_prediction_without_delays/Prediction_and_cost_function1/Subsystem/Subsystem2/Add1 ==
  In1 : Inport
  In2 : Inport  Port=2
  Add1 : Sum  OutDataTypeStr=single  SampleTime=1e-08
  Add1_pd1 : Delay  DelayLength=6
  Out1 : Outport
  wires:
  In1/1 -> Add1/1
  In2/1 -> Add1/2
  Add1/1 -> Add1_pd1/1
  Add1_pd1/1 -> Out1/1

== system gm_test_prediction_without_delays/Prediction_and_cost_function1/Subsystem/Subsystem2/Add2 ==
  In1 : Inport
  In2 : Inport  Port=2
  Add2 : Sum  OutDataTypeStr=single  SampleTime=1e-08
  Add2_pd1 : Delay  DelayLength=6
  Out1 : Outport
  wires:
  In1/1 -> Add2/1
  In2/1 -> Add2/2
  Add2/1 -> Add2_pd1/1
  Add2_pd1/1 -> Out1/1

== system gm_test_prediction_without_delays/Prediction_and_cost_function1/Subsystem/Subsystem2/Add3 ==
  In1 : Inport
  In2 : Inport  Port=2
  Add3 : Sum  OutDataTypeStr=single  SampleTime=1e-08
  Add3_pd1 : Delay  DelayLength=6
  Out1 : Outport
  wires:
  In1/1 -> Add3/1
  In2/1 -> Add3/2
  Add3/1 -> Add3_pd1/1
  Add3_pd1/1 -> Out1/1

== system gm_test_prediction_without_delays/Prediction_and_cost_function1/Subsystem/Subsystem2/Add4 ==
  In1 : Inport
  In2 : Inport  Port=2
  Add4 : Sum  OutDataTypeStr=single  SampleTime=1e-08
  Add4_pd1 : Delay  DelayLength=6
  Out1 : Outport
  wires:
  In1/1 -> Add4/1
  In2/1 -> Add4/2
  Add4/1 -> Add4_pd1/1
  Add4_pd1/1 -> Out1/1

== system gm_test_prediction_without_delays/Prediction_and_cost_function1/Subsystem/Subsystem2/Product1 ==
  In1 : Inport
  In2 : Inport  Port=2
  Product1 : Product  Inputs=**  OutDataTypeStr=single  SampleTime=1e-08
  Product1_pd1 : Delay  DelayLength=6
  Out1 : Outport
  wires:
  In1/1 -> Product1/1
  In2/1 -> Product1/2
  Product1/1 -> Product1_pd1/1
  Product1_pd1/1 -> Out1/1

== system gm_test_prediction_without_delays/Prediction_and_cost_function1/Subsystem/Subsystem2/Product10 ==
  In1 : Inport
  In2 : Inport  Port=2
  Product10 : Product  Inputs=**  OutDataTypeStr=single  SampleTime=1e-08
  Product10_pd1 : Delay  DelayLength=6
  Out1 : Outport
  wires:
  In1/1 -> Product10/1
  In2/1 -> Product10/2
  Product10/1 -> Product10_pd1/1
  Product10_pd1/1 -> Out1/1

== system gm_test_prediction_without_delays/Prediction_and_cost_function1/Subsystem/Subsystem2/Product11 ==
  In1 : Inport
  In2 : Inport  Port=2
  Product11 : Product  Inputs=**  OutDataTypeStr=single  SampleTime=1e-08
  Product11_pd1 : Delay  DelayLength=6
  Out1 : Outport
  wires:
  In1/1 -> Product11/1
  In2/1 -> Product11/2
  Product11/1 -> Product11_pd1/1
  Product11_pd1/1 -> Out1/1

== system gm_test_prediction_without_delays/Prediction_and_cost_function1/Subsystem/Subsystem2/Product2 ==
  In1 : Inport
  In2 : Inport  Port=2
  Product2 : Product  Inputs=**  OutDataTypeStr=single  SampleTime=1e-08
  Product2_pd1 : Delay  DelayLength=6
  Out1 : Outport
  wires:
  In1/1 -> Product2/1
  In2/1 -> Product2/2
  Product2/1 -> Product2_pd1/1
  Product2_pd1/1 -> Out1/1

== system gm_test_prediction_without_delays/Prediction_and_cost_function1/Subsystem/Subsystem2/Product3 ==
  In1 : Inport
  In2 : Inport  Port=2
  Product3 : Product  Inputs=**  OutDataTypeStr=single  SampleTime=1e-08
  Product3_pd1 : Delay  DelayLength=6
  Out1 : Outport
  wires:
  In1/1 -> Product3/1
  In2/1 -> Product3/2
  Product3/1 -> Product3_pd1/1
  Product3_pd1/1 -> Out1/1

== system gm_test_prediction_without_delays/Prediction_and_cost_function1/Subsystem/Subsystem2/Product31 ==
  In1 : Inport
  In2 : Inport  Port=2
  Product31 : Product  Inputs=**  OutDataTypeStr=single  SampleTime=1e-08
  Product31_pd1 : Delay  DelayLength=6
  Out1 : Outport
  wires:
  In1/1 -> Product31/1
  In2/1 -> Product31/2
  Product31/1 -> Product31_pd1/1
  Product31_pd1/1 -> Out1/1

== system gm_test_prediction_without_delays/Prediction_and_cost_function1/Subsystem/Subsystem2/Product4 ==
  In1 : Inport
  In2 : Inport  Port=2
  Product4 : Product  Inputs=**  OutDataTypeStr=single  SampleTime=1e-08
  Product4_pd1 : Delay  DelayLength=6
  Out1 : Outport
  wires:
  In1/1 -> Product4/1
  In2/1 -> Product4/2
  Product4/1 -> Product4_pd1/1
  Product4_pd1/1 -> Out1/1

== system gm_test_prediction_without_delays/Prediction_and_cost_function1/Subsystem/Subsystem2/Product5 ==
  In1 : Inport
  In2 : Inport  Port=2
  Product5 : Product  Inputs=**  OutDataTypeStr=single  SampleTime=1e-08
  Product5_pd1 : Delay  DelayLength=6
  Out1 : Outport
  wires:
  In1/1 -> Product5/1
  In2/1 -> Product5/2
  Product5/1 -> Product5_pd1/1
  Product5_pd1/1 -> Out1/1

== system gm_test_prediction_without_delays/Prediction_and_cost_function1/Subsystem/Subsystem2/Product6 ==
  In1 : Inport
  In2 : Inport  Port=2
  Product6 : Product  Inputs=**  OutDataTypeStr=single  SampleTime=1e-08
  Product6_pd1 : Delay  DelayLength=6
  Out1 : Outport
  wires:
  In1/1 -> Product6/1
  In2/1 -> Product6/2
  Product6/1 -> Product6_pd1/1
  Product6_pd1/1 -> Out1/1

== system gm_test_prediction_without_delays/Prediction_and_cost_function1/Subsystem/Subsystem2/Product7 ==
  In1 : Inport
  In2 : Inport  Port=2
  Product7 : Product  Inputs=**  OutDataTypeStr=single  SampleTime=1e-08
  Product7_pd1 : Delay  DelayLength=6
  Out1 : Outport
  wires:
  In1/1 -> Product7/1
  In2/1 -> Product7/2
  Product7/1 -> Product7_pd1/1
  Product7_pd1/1 -> Out1/1

== system gm_test_prediction_without_delays/Prediction_and_cost_function1/Subsystem/Subsystem2/Product8 ==
  In1 : Inport
  In2 : Inport  Port=2
  Product8 : Product  Inputs=**  OutDataTypeStr=single  SampleTime=1e-08
  Product8_pd1 : Delay  DelayLength=6
  Out1 : Outport
  wires:
  In1/1 -> Product8/1
  In2/1 -> Product8/2
  Product8/1 -> Product8_pd1/1
  Product8_pd1/1 -> Out1/1

== system gm_test_prediction_without_delays/Prediction_and_cost_function1/Subsystem/Subsystem2/Product9 ==
  In1 : Inport
  In2 : Inport  Port=2
  Product9 : Product  Inputs=**  OutDataTypeStr=single  SampleTime=1e-08
  Product9_pd1 : Delay  DelayLength=6
  Out1 : Outport
  wires:
  In1/1 -> Product9/1
  In2/1 -> Product9/2
  Product9/1 -> Product9_pd1/1
  Product9_pd1/1 -> Out1/1

== system gm_test_prediction_without_delays/Prediction_and_cost_function1/Subsystem/Subsystem2/Subtract1_stage2 ==
  In1 : Inport
  In2 : Inport  Port=2
  Subtract1_stage2 : Sum  Inputs=+-  OutDataTypeStr=single  SampleTime=1e-08
  Subtract1_stage2_pd1 : Delay  DelayLength=6
  Out1 : Outport
  wires:
  In1/1 -> Subtract1_stage2/1
  In2/1 -> Subtract1_stage2/2
  Subtract1_stage2/1 -> Subtract1_stage2_pd1/1
  Subtract1_stage2_pd1/1 -> Out1/1

== system gm_test_prediction_without_delays/Prediction_and_cost_function1/Subsystem/Subsystem2/Subtract1_stage3 ==
  In1 : Inport
  In2 : Inport  Port=2
  Subtract1_stage3 : Sum  Inputs=+-  OutDataTypeStr=single  SampleTime=1e-08
  Subtract1_stage3_pd1 : Delay  DelayLength=6
  Out1 : Outport
  wires:
  In1/1 -> Subtract1_stage3/1
  In2/1 -> Subtract1_stage3/2
  Subtract1_stage3/1 -> Subtract1_stage3_pd1/1
  Subtract1_stage3_pd1/1 -> Out1/1

== system gm_test_prediction_without_delays/Prediction_and_cost_function1/Subsystem/Subsystem2/Subtract2 ==
  In1 : Inport
  In2 : Inport  Port=2
  Subtract2 : Sum  Inputs=+-  OutDataTypeStr=single  SampleTime=1e-08
  Subtract2_pd1 : Delay  DelayLength=6
  Out1 : Outport
  wires:
  In1/1 -> Subtract2/1
  In2/1 -> Subtract2/2
  Subtract2/1 -> Subtract2_pd1/1
  Subtract2_pd1/1 -> Out1/1

== system gm_test_prediction_without_delays/Prediction_and_cost_function1/Subsystem/Subsystem2/Subtract3 ==
  In1 : Inport
  In2 : Inport  Port=2
  Subtract3 : Sum  Inputs=+-  OutDataTypeStr=single  SampleTime=1e-08
  Subtract3_pd1 : Delay  DelayLength=6
  Out1 : Outport
  wires:
  In1/1 -> Subtract3/1
  In2/1 -> Subtract3/2
  Subtract3/1 -> Subtract3_pd1/1
  Subtract3_pd1/1 -> Out1/1

== system gm_test_prediction_without_delays/Prediction_and_cost_function1/Subsystem/Subsystem2/Subtract_stage2 ==
  In1 : Inport
  In2 : Inport  Port=2
  Subtract_stage2 : Sum  Inputs=+-  OutDataTypeStr=single  SampleTime=1e-08
  Subtract_stage2_pd1 : Delay  DelayLength=6
  Out1 : Outport
  wires:
  In1/1 -> Subtract_stage2/1
  In2/1 -> Subtract_stage2/2
  Subtract_stage2/1 -> Subtract_stage2_pd1/1
  Subtract_stage2_pd1/1 -> Out1/1

== system gm_test_prediction_without_delays/Prediction_and_cost_function1/Subsystem/Subsystem2/Subtract_stage3 ==
  In1 : Inport
  In2 : Inport  Port=2
  Subtract_stage3 : Sum  OutDataTypeStr=single  SampleTime=1e-08
  Subtract_stage3_pd1 : Delay  DelayLength=6
  Out1 : Outport
  wires:
  In1/1 -> Subtract_stage3/1
  In2/1 -> Subtract_stage3/2
  Subtract_stage3/1 -> Subtract_stage3_pd1/1
  Subtract_stage3_pd1/1 -> Out1/1

== system gm_test_prediction_without_delays/Prediction_and_cost_function1/Subsystem/Subsystem3/Add ==
  In1 : Inport
  In2 : Inport  Port=2
  Add : Sum  OutDataTypeStr=single  SampleTime=1e-08
  Add_pd1 : Delay  DelayLength=6
  Out1 : Outport
  wires:
  In1/1 -> Add/1
  In2/1 -> Add/2
  Add/1 -> Add_pd1/1
  Add_pd1/1 -> Out1/1

== system gm_test_prediction_without_delays/Prediction_and_cost_function1/Subsystem/Subsystem3/Add1 ==
  In1 : Inport
  In2 : Inport  Port=2
  Add1 : Sum  OutDataTypeStr=single  SampleTime=1e-08
  Add1_pd1 : Delay  DelayLength=6
  Out1 : Outport
  wires:
  In1/1 -> Add1/1
  In2/1 -> Add1/2
  Add1/1 -> Add1_pd1/1
  Add1_pd1/1 -> Out1/1

== system gm_test_prediction_without_delays/Prediction_and_cost_function1/Subsystem/Subsystem3/Add2 ==
  In1 : Inport
  In2 : Inport  Port=2
  Add2 : Sum  OutDataTypeStr=single  SampleTime=1e-08
  Add2_pd1 : Delay  DelayLength=6
  Out1 : Outport
  wires:
  In1/1 -> Add2/1
  In2/1 -> Add2/2
  Add2/1 -> Add2_pd1/1
  Add2_pd1/1 -> Out1/1

== system gm_test_prediction_without_delays/Prediction_and_cost_function1/Subsystem/Subsystem3/Add3 ==
  In1 : Inport
  In2 : Inport  Port=2
  Add3 : Sum  OutDataTypeStr=single  SampleTime=1e-08
  Add3_pd1 : Delay  DelayLength=6
  Out1 : Outport
  wires:
  In1/1 -> Add3/1
  In2/1 -> Add3/2
  Add3/1 -> Add3_pd1/1
  Add3_pd1/1 -> Out1/1

== system gm_test_prediction_without_delays/Prediction_and_cost_function1/Subsystem/Subsystem3/Add4 ==
  In1 : Inport
  In2 : Inport  Port=2
  Add4 : Sum  OutDataTypeStr=single  SampleTime=1e-08
  Add4_pd1 : Delay  DelayLength=6
  Out1 : Outport
  wires:
  In1/1 -> Add4/1
  In2/1 -> Add4/2
  Add4/1 -> Add4_pd1/1
  Add4_pd1/1 -> Out1/1

== system gm_test_prediction_without_delays/Prediction_and_cost_function1/Subsystem/Subsystem3/Product1 ==
  In1 : Inport
  In2 : Inport  Port=2
  Product1 : Product  Inputs=**  OutDataTypeStr=single  SampleTime=1e-08
  Product1_pd1 : Delay  DelayLength=6
  Out1 : Outport
  wires:
  In1/1 -> Product1/1
  In2/1 -> Product1/2
  Product1/1 -> Product1_pd1/1
  Product1_pd1/1 -> Out1/1

== system gm_test_prediction_without_delays/Prediction_and_cost_function1/Subsystem/Subsystem3/Product10 ==
  In1 : Inport
  In2 : Inport  Port=2
  Product10 : Product  Inputs=**  OutDataTypeStr=single  SampleTime=1e-08
  Product10_pd1 : Delay  DelayLength=6
  Out1 : Outport
  wires:
  In1/1 -> Product10/1
  In2/1 -> Product10/2
  Product10/1 -> Product10_pd1/1
  Product10_pd1/1 -> Out1/1

== system gm_test_prediction_without_delays/Prediction_and_cost_function1/Subsystem/Subsystem3/Product11 ==
  In1 : Inport
  In2 : Inport  Port=2
  Product11 : Product  Inputs=**  OutDataTypeStr=single  SampleTime=1e-08
  Product11_pd1 : Delay  DelayLength=6
  Out1 : Outport
  wires:
  In1/1 -> Product11/1
  In2/1 -> Product11/2
  Product11/1 -> Product11_pd1/1
  Product11_pd1/1 -> Out1/1

== system gm_test_prediction_without_delays/Prediction_and_cost_function1/Subsystem/Subsystem3/Product2 ==
  In1 : Inport
  In2 : Inport  Port=2
  Product2 : Product  Inputs=**  OutDataTypeStr=single  SampleTime=1e-08
  Product2_pd1 : Delay  DelayLength=6
  Out1 : Outport
  wires:
  In1/1 -> Product2/1
  In2/1 -> Product2/2
  Product2/1 -> Product2_pd1/1
  Product2_pd1/1 -> Out1/1

== system gm_test_prediction_without_delays/Prediction_and_cost_function1/Subsystem/Subsystem3/Product3 ==
  In1 : Inport
  In2 : Inport  Port=2
  Product3 : Product  Inputs=**  OutDataTypeStr=single  SampleTime=1e-08
  Product3_pd1 : Delay  DelayLength=6
  Out1 : Outport
  wires:
  In1/1 -> Product3/1
  In2/1 -> Product3/2
  Product3/1 -> Product3_pd1/1
  Product3_pd1/1 -> Out1/1

== system gm_test_prediction_without_delays/Prediction_and_cost_function1/Subsystem/Subsystem3/Product31 ==
  In1 : Inport
  In2 : Inport  Port=2
  Product31 : Product  Inputs=**  OutDataTypeStr=single  SampleTime=1e-08
  Product31_pd1 : Delay  DelayLength=6
  Out1 : Outport
  wires:
  In1/1 -> Product31/1
  In2/1 -> Product31/2
  Product31/1 -> Product31_pd1/1
  Product31_pd1/1 -> Out1/1

== system gm_test_prediction_without_delays/Prediction_and_cost_function1/Subsystem/Subsystem3/Product4 ==
  In1 : Inport
  In2 : Inport  Port=2
  Product4 : Product  Inputs=**  OutDataTypeStr=single  SampleTime=1e-08
  Product4_pd1 : Delay  DelayLength=6
  Out1 : Outport
  wires:
  In1/1 -> Product4/1
  In2/1 -> Product4/2
  Product4/1 -> Product4_pd1/1
  Product4_pd1/1 -> Out1/1

== system gm_test_prediction_without_delays/Prediction_and_cost_function1/Subsystem/Subsystem3/Product5 ==
  In1 : Inport
  In2 : Inport  Port=2
  Product5 : Product  Inputs=**  OutDataTypeStr=single  SampleTime=1e-08
  Product5_pd1 : Delay  DelayLength=6
  Out1 : Outport
  wires:
  In1/1 -> Product5/1
  In2/1 -> Product5/2
  Product5/1 -> Product5_pd1/1
  Product5_pd1/1 -> Out1/1

== system gm_test_prediction_without_delays/Prediction_and_cost_function1/Subsystem/Subsystem3/Product6 ==
  In1 : Inport
  In2 : Inport  Port=2
  Product6 : Product  Inputs=**  OutDataTypeStr=single  SampleTime=1e-08
  Product6_pd1 : Delay  DelayLength=6
  Out1 : Outport
  wires:
  In1/1 -> Product6/1
  In2/1 -> Product6/2
  Product6/1 -> Product6_pd1/1
  Product6_pd1/1 -> Out1/1

== system gm_test_prediction_without_delays/Prediction_and_cost_function1/Subsystem/Subsystem3/Product7 ==
  In1 : Inport
  In2 : Inport  Port=2
  Product7 : Product  Inputs=**  OutDataTypeStr=single  SampleTime=1e-08
  Product7_pd1 : Delay  DelayLength=6
  Out1 : Outport
  wires:
  In1/1 -> Product7/1
  In2/1 -> Product7/2
  Product7/1 -> Product7_pd1/1
  Product7_pd1/1 -> Out1/1

== system gm_test_prediction_without_delays/Prediction_and_cost_function1/Subsystem/Subsystem3/Product8 ==
  In1 : Inport
  In2 : Inport  Port=2
  Product8 : Product  Inputs=**  OutDataTypeStr=single  SampleTime=1e-08
  Product8_pd1 : Delay  DelayLength=6
  Out1 : Outport
  wires:
  In1/1 -> Product8/1
  In2/1 -> Product8/2
  Product8/1 -> Product8_pd1/1
  Product8_pd1/1 -> Out1/1
